simulink model "the_pid"  (R2019b)
settings: Solver=VariableStepAuto  StartTime=0.0  StopTime=10.0  RelTol=1e-3
values from neighbouring files (symbols this model uses):
  Kd = 50    [damper_pid_run.m]    (also in pid_tune_run.m = 2.438)
  Ki = 40    [adaptive_cruise.m]    (also in damper_pid_run.m = 300; pid_tune_run.m = 114.7)
  Kp = 800    [adaptive_cruise.m]    (also in damper_pid_run.m = 350; pid_tune_run.m = 37.8)
settings Model: Creator=dgander  LastModifiedBy=dgander

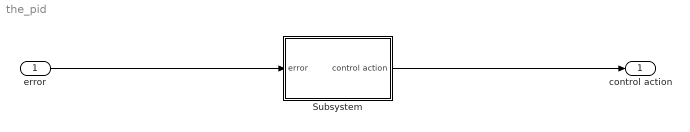
== system the_pid ==
  error : Inport
  Subsystem : Subsystem
  control action : Outport
  wires:
  error/1 -> Subsystem/1(error)
  Subsystem/1(control action) -> control action/1

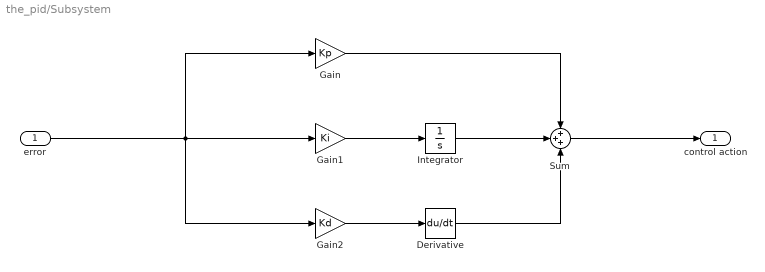
== system the_pid/Subsystem ==
  error : Inport
  Derivative : Derivative
  Gain : Gain  Gain=Kp
  Gain1 : Gain  Gain=Ki
  Gain2 : Gain  Gain=Kd
  Integrator : Integrator
  Sum : Sum  Inputs=+++
  control action : Outport
  wires:
  Gain1/1 -> Integrator/1
  Sum/1 -> control action/1
  Integrator/1 -> Sum/2
  error/1 -> Gain2/1, Gain1/1, Gain/1
  Gain/1 -> Sum/1
  Derivative/1 -> Sum/3
  Gain2/1 -> Derivative/1
